simulink model "gainSchedExample_nonlinPlant_nonlinCntr"  (R2020b)
settings: Solver=VariableStepAuto  StartTime=0.0  StopTime=10.0  MinStep=TSim/5000  RelTol=1e-3
values from neighbouring files (symbols this model uses):
  cntr =     [cntrDesign_1.mat]    (also in cntrDesign_2.mat)
  initVal = 1    [Run_AcademicExample.m]
  refVal = 1.5    [Run_AcademicExample.m]
  tStep = 3.5    [Run_AcademicExample.m]
  umax = 8    [Design_ControllerObserverAndAW.m]    (also in Run_AcademicExample.m = 800)
  xInit = cntr.xAP_1    [Design_ControllerObserverAndAW.m]    (also in Run_AcademicExample.m)
undefined symbols (not defined in the file or in its folder): system
settings Model: Creator=Kefferpuetz  LastModifiedBy=Kefferpuetz

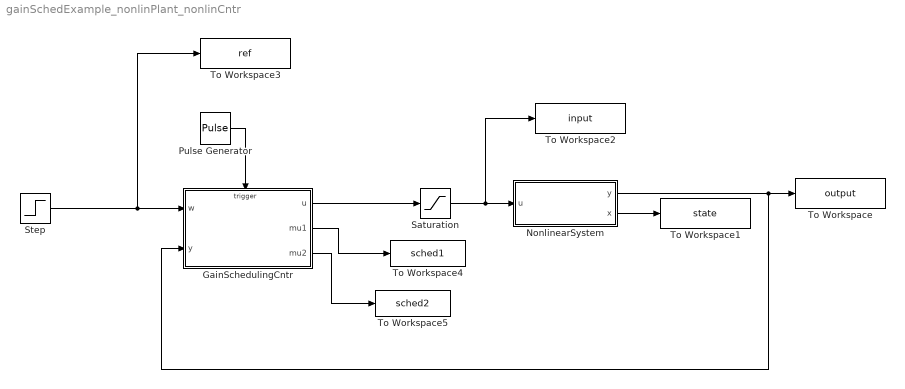
== system gainSchedExample_nonlinPlant_nonlinCntr ==
  GainSchedulingCntr : Subsystem
  NonlinearSystem : Subsystem
  Pulse Generator : DiscretePulseGenerator  PulseType=Time based  Period=cntr.TS  PulseWidth=50
  Saturation : Saturate  UpperLimit=umax  LowerLimit=-umax
  Step : Step  Time=tStep  Before=initVal  After=refVal  SampleTime=0
  To Workspace : ToWorkspace  VariableName=output  SaveFormat=Structure With Time  SampleTime=-1
  To Workspace1 : ToWorkspace  VariableName=state  SaveFormat=Structure With Time  SampleTime=-1
  To Workspace2 : ToWorkspace  VariableName=input  SaveFormat=Structure With Time  SampleTime=-1
  To Workspace3 : ToWorkspace  VariableName=ref  SaveFormat=Structure With Time  SampleTime=-1
  To Workspace4 : ToWorkspace  VariableName=sched1  SaveFormat=Structure With Time  SampleTime=-1
  To Workspace5 : ToWorkspace  VariableName=sched2  SaveFormat=Structure With Time  SampleTime=-1
  wires:
  NonlinearSystem/2(x) -> To Workspace1/1
  NonlinearSystem/1(y) -> GainSchedulingCntr/2(y), To Workspace/1
  GainSchedulingCntr/1(u) -> Saturation/1
  Saturation/1 -> To Workspace2/1, NonlinearSystem/1(u)
  Step/1 -> To Workspace3/1, GainSchedulingCntr/1(w)
  Pulse Generator/1 -> GainSchedulingCntr/Trigger
  GainSchedulingCntr/2(mu1) -> To Workspace4/1
  GainSchedulingCntr/3(mu2) -> To Workspace5/1

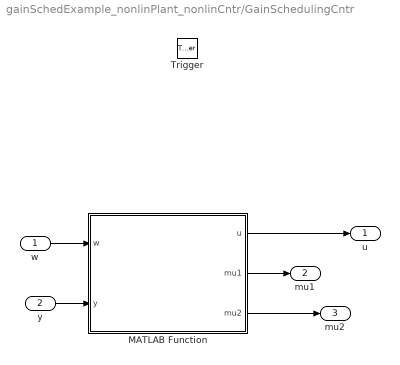
== system gainSchedExample_nonlinPlant_nonlinCntr/GainSchedulingCntr ==
  w : Inport
  y : Inport  Port=2
  Trigger : TriggerPort  VariantControl=Variant  PortDimensions=1
  MATLAB Function : MATLAB Function  TreatAsAtomicUnit=on
  u : Outport
  mu1 : Outport  Port=2
  mu2 : Outport  Port=3
  wires:
  MATLAB Function/1(u) -> u/1
  y/1 -> MATLAB Function/2(y)
  w/1 -> MATLAB Function/1(w)
  MATLAB Function/2(mu1) -> mu1/1
  MATLAB Function/3(mu2) -> mu2/1

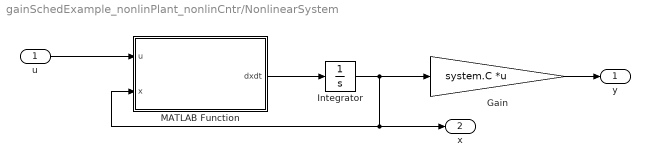
== system gainSchedExample_nonlinPlant_nonlinCntr/NonlinearSystem ==
  u : Inport
  Gain : Gain  Gain=system.C  Multiplication=Matrix(K*u) (u vector)
  Integrator : Integrator  InitialCondition=xInit
  MATLAB Function : MATLAB Function  TreatAsAtomicUnit=on
  y : Outport
  x : Outport  Port=2
  wires:
  Gain/1 -> y/1
  Integrator/1 -> Gain/1, MATLAB Function/2(x), x/1
  MATLAB Function/1(dxdt) -> Integrator/1
  u/1 -> MATLAB Function/1(u)

== matlab function gainSchedExample_nonlinPlant_nonlinCntr/GainSchedulingCntr/MATLAB Function ==
  data: w input; y input; u output; cntr parameter; mu1 output; mu2 output
function [u, mu1, mu2]  = gainSchedulingCntr( w, y,  cntr)
  % This function implements a discretized version of a gain-scheduling  
  % controller designed to work in between two operating points
  % The controller relies on control signal blending and requires an
  % anti-windup to operate reliable/without performance degradations
  % However, anti-windup can be deactivated setting cntr.awOn = 0
  %
  %
  % Author: Klaus Kefferpütz, University of Applied Sciences Augsburg 2021
  % email: klaus.kefferpuetz@hs-augsburg.de 
  persistent xI_1;
  persistent xI_2;
  persistent xAW_1;
  persistent xAW_2;
  persistent xEst_1;
  persistent xEst_2;
  
  if(isempty(xI_1))
     xI_1 = 0;
     xI_2 = 0;
     xAW_1 = zeros(2,1);
     xAW_2 = zeros(2,1);
     xEst_1 = zeros(2,1);
     xEst_2 = zeros(2,1);
  end

  TS = cntr.TS;
  
  % compute affiliation function values for current y (here p=y)
  % p is constrained to vary between xAP(1) and xAP(2) since
  % we have to incorporate more controllers to operate below xAP(1)
  % and above xAP(2)
  if(y>cntr.xAP_2(1))
    p = cntr.xAP_2(1);
    mu1 = 0;
    mu2 = 1;
  elseif (y<cntr.xAP_1(1)) 
    p = cntr.xAP_1(1);
    mu1 = 1;
    mu2 = 0;
  else
    p = y; 
    % in between our operating points  p1<p<p_2
    mu1 = 0.5*(1+cos(pi*(p-cntr.xAP_1(1))/(cntr.xAP_2(1)-cntr.xAP_1(1)) ) );
    mu2 = 0.5*(1-cos(pi*(p-cntr.xAP_1(1))/(cntr.xAP_2(1)-cntr.xAP_1(1)) ) );
  end


  % only if anti-windup is activated, i.e. cntr.awOn = 1
  if(cntr.awOn)
      % compute AW outputs
      yawu_1 = -cntr.CAW*xAW_1;
      yawy_1 = -cntr.Kaw1*xAW_1;
      yawu_2 = -cntr.CAW*xAW_2;
      yawy_2 = -cntr.Kaw2*xAW_2;
      % compute controller inputs
      y1 = y-yawu_1;
      y2 = y-yawu_2;
  else
      yawu_1 = 0;
      yawu_2 = 0;
      yawy_1 = 0;
      yawy_2 = 0;
  
      % compute controller inputs without anti-windup
      y1 = y;
      y2 = y;
  end
  yAP_1 = cntr.xAP_1(1);
  yAP_2 = cntr.xAP_2(1);
  
  delta_y1 = y1-yAP_1;
  delta_y2 = y2-yAP_2;
  %_____________________________________________________________________
  % Update PI-state space control law
  u_1   = cntr.Kp1*(w-y1)+cntr.Ki1*xI_1-cntr.K_1*xEst_1+cntr.uAP_1;
  u_2   = cntr.Kp2*(w-y2)+cntr.Ki2*xI_2-cntr.K_2*xEst_2+cntr.uAP_2;

  % update integrator state of PI state space controller
  xI_1 = xI_1+TS*(w-y1);
  xI_2 = xI_2+TS*(w-y2);
  
  % perform control signal blending
  if(cntr.awOn)
    % in case anti-windup is active, controller output is modified  
    uTotal = mu1*(u_1+yawy_1)+mu2*(u_2+yawy_2);
  else
    % just blending in case now anti-windup active  
    uTotal = mu1*u_1+mu2*u_2;  
  end
  
  %_____________________________________________________________________
  % Update linear observer 
  yEst_1     = cntr.C*xEst_1;
  % providing the actual (blended & saturated control signal should minimize the risk of estimation errors, but 
  % you might also use the commented version instead but it will tend to increase the risk of blending/saturation induced windup 
  % further making MRAW even more beneficial.
  xEst_kP_1  = xEst_1 + TS*( cntr.A1*xEst_1+cntr.B1*(sat(uTotal, cntr.umax)-cntr.uAP_1)+cntr.L1*(delta_y1-yEst_1));  
  % xEst_kP_1  = xEst_1 + TS*( cntr.A1*xEst_1+cntr.B1*(u_1-cntr.uAP_1)+cntr.L1*(delta_y1-yEst_1)); 
  xEst_1     = xEst_kP_1;
   
  yEst_2     = cntr.C*xEst_2;
  % providing the actual (blended & saturated control signal should minimize the risk of estimation errors, but 
  % you might also use the commented version instead)
  xEst_kP_2  = xEst_2 + TS*( cntr.A2*xEst_2+cntr.B2*(sat(uTotal, cntr.umax)-cntr.uAP_2)+cntr.L2*(delta_y2-yEst_2));  
  % xEst_kP_2  = xEst_2 + TS*( cntr.A2*xEst_2+cntr.B2*(u_2-cntr.uAP_2)+cntr.L2*(delta_y2-yEst_2));  
  xEst_2     = xEst_kP_2;
  
  %_____________________________________________________________________
  % compute AW inputs, difference between controller command u_i and
  % actually realized control signal uTotal (affected by blending)
  deltaIn_1    = u_1-sat(uTotal, cntr.umax);
  deltaIn_2    = u_2-sat(uTotal, cntr.umax);
  
  % update AW networks of each controller
  xAW_1_new = xAW_1 + TS*((cntr.A1*mu1+cntr.A2*mu2)*xAW_1+(cntr.B1*mu1+cntr.B2*mu2)*deltaIn_1);
  xAW_1     = xAW_1_new;
  
  xAW_2_new = xAW_2 + TS*((cntr.A1*mu1+cntr.A2*mu2)*xAW_2+(cntr.B1*mu1+cntr.B2*mu2)*deltaIn_2);
  xAW_2     = xAW_2_new;
  
  u = uTotal;

== matlab function gainSchedExample_nonlinPlant_nonlinCntr/NonlinearSystem/MATLAB Function ==
  data: u input; x input; dxdt output
function dxdt  = fcn(u, x)
    dxdt = zeros(2,1);    

    
   
    dxdt(1) = x(2);
    dxdt(2) = x(1)*(1-x(2))+u;
